simulink model "Antenna_Positioner_simulation"  (R2023b)
settings: Solver=VariableStepAuto  StartTime=0.0  StopTime=10.0  RelTol=1e-3  EnableMultiTasking=on
settings Model: Creator=acesxx  LastModifiedBy=avikd
settings SolverCC: AlgebraicLoopSolver=TrustRegion
settings DataIOCC: ReturnWorkspaceOutputs=off
settings OptimizationCC: LifeSpan=inf
settings DebuggingCC: UnconnectedInputMsg=warning  UnconnectedOutputMsg=warning  UnconnectedLineMsg=warning  SFUnexpectedBacktrackingDiag=warning  SFNoUnconditionalDefaultTransitionDiag=warning  ArithmeticOperatorsInVariantConditions=warning
settings ModelReferenceCC: EnableRefExpFcnMdlSchedulingChecks=on
settings SFSimCC: SimUseLocalCustomCode=off  CustomCodeUndefinedFunction=UseInterfaceOnly
settings RTWCC: RTWUseLocalCustomCode=off
settings CodeAppCC: StateflowObjectComments=on
settings GRTTargetCC: TargetLangStandard=C89/C90 (ANSI)
settings ConfigComp: CovMetricSettings=dw  CovSaveCumulativeToWorkspaceVar=on  CovSaveSingleToWorkspaceVar=on  CovExternalEMLEnable=off

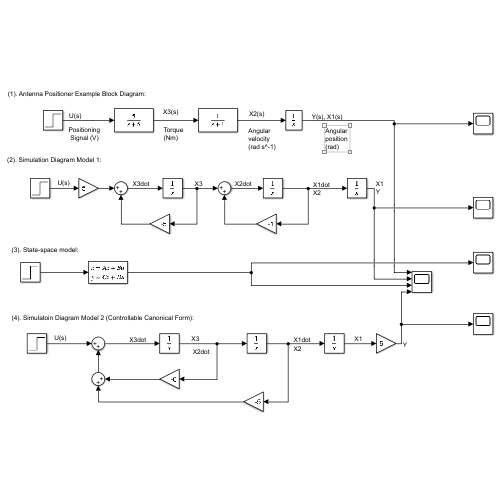
[thumbnail: Simulink's stored preview of the top-level diagram]
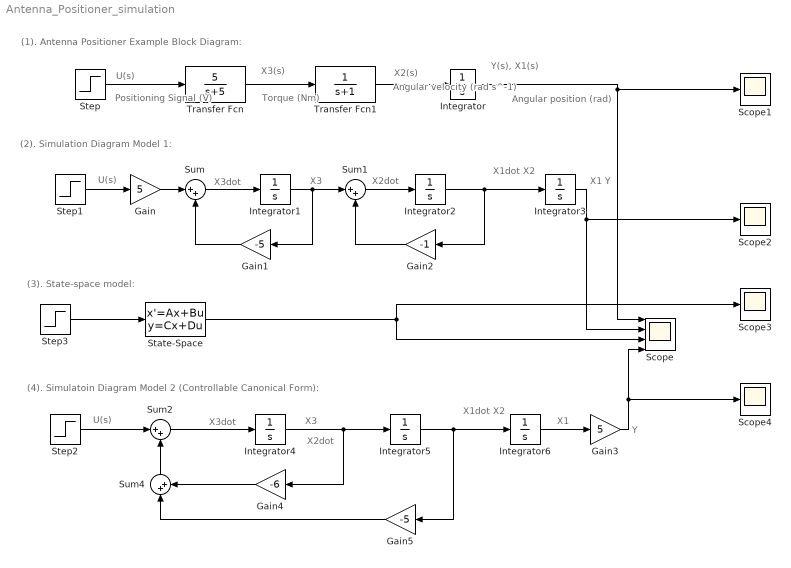
== system Antenna_Positioner_simulation ==
  note: (3). State-space model:
  note: Y
  note: X1
  note: X1
      | Y
  note: X1dot
      | X2
  note: X2dot
  note: X3
  note: X3dot
  note: U(s)
  note: Angular
      | position
      | (rad)
  note: Angular
      | velocity
      | (rad s^-1)
  note: Torque
      | (Nm)
  note: Positioning
      |  Signal (V)
  note: U(s)
  note: X3(s)
  note: X2(s)
  note: Y(s), X1(s)
  note: (4). Simulatoin Diagram Model 2 (Controllable Canonical Form):
  note: (2). Simulation Diagram Model 1:
  note: (1). Antenna Positioner Example Block Diagram:
  note: X1dot
      | X2
  note: X2dot
  note: X3
  note: X3dot
  note: U(s)
  Gain : Gain  Gain=5
  Gain1 : Gain  Gain=-5
  Gain2 : Gain  Gain=-1
  Gain3 : Gain  Gain=5
  Gain4 : Gain  Gain=-6
  Gain5 : Gain  Gain=-5
  Integrator{,1..6} (7 alike) : Integrator
  Scope : Scope  NumInputPorts=4
  Scope{1..4} (4 alike) : Scope
  State-Space : StateSpace  A=[0 1 0; 0 -1 1; 0 0 -5]  B=[0;0;5]  C=[1 0 0]  D=0  InitialCondition=0
  Step{,1..3} (4 alike) : Step  SampleTime=0
  Sum{,1..2,4} (4 alike) : Sum  Inputs=|++
  Transfer Fcn : TransferFcn  Numerator=[5]  Denominator=[1 5]
  Transfer Fcn1 : TransferFcn  Denominator=[1 1]
  wires:
  Step/1 -> Transfer Fcn/1
  Transfer Fcn/1 -> Transfer Fcn1/1
  Transfer Fcn1/1 -> Integrator/1
  Integrator/1 -> Scope1/1, Scope/1
  Step1/1 -> Gain/1
  Gain/1 -> Sum/1
  Sum/1 -> Integrator1/1
  Integrator1/1 -> Gain1/1, Sum1/1
  Gain1/1 -> Sum/2
  Sum1/1 -> Integrator2/1
  Integrator2/1 -> Gain2/1, Integrator3/1
  Gain2/1 -> Sum1/2
  Integrator3/1 -> Scope2/1, Scope/2
  Step2/1 -> Sum2/1
  Sum2/1 -> Integrator4/1
  Integrator5/1 -> Gain5/1, Integrator6/1
  Sum4/1 -> Sum2/2
  Integrator4/1 -> Gain4/1, Integrator5/1
  Gain5/1 -> Sum4/1
  Gain4/1 -> Sum4/2
  Integrator6/1 -> Gain3/1
  Step3/1 -> State-Space/1
  State-Space/1 -> Scope3/1, Scope/3
  Gain3/1 -> Scope4/1, Scope/4
